simulink model "SF005A_StOutpCtrl"  (R2013b)
settings: Solver=FixedStepDiscrete  SolverMode=SingleTasking  StartTime=0.0  StopTime=1  FixedStep=0.002  RelTol=1e-3
values from neighbouring files (symbols this model uses):
  ARCHGLBPRM_2MILLISEC_SEC_F32 = DataDict.Constant    [SF005A_StOutpCtrl_DataDict.m]
  ARCHGLBPRM_FLOATZEROTHD_ULS_F32 = DataDict.Constant    [SF005A_StOutpCtrl_DataDict.m]
  BIGSLEW_ULSPERSEC_F32 = DataDict.Constant    [SF005A_StOutpCtrl_DataDict.m]
  DI_CNT_U08 = DataDict.Constant    [SF005A_StOutpCtrl_DataDict.m]
  LOA_CNT_U08 = DataDict.Constant    [SF005A_StOutpCtrl_DataDict.m]
  OPER_CNT_U08 = DataDict.Constant    [SF005A_StOutpCtrl_DataDict.m]
  STRTSTOP_CNT_U08 = DataDict.Constant    [SF005A_StOutpCtrl_DataDict.m]
libraries: NxtrLim x3, simulink x2
(part 1 of 2)
settings Model: Creator=lzz0tm  LastModifiedBy=FZG88Y
settings SolverCC: AutoInsertRateTranBlk=on  InsertRTBMode=Always
settings DataIOCC: LimitDataPoints=off  SaveFormat=Structure  ReturnWorkspaceOutputs=on
settings OptimizationCC: BlockReduction=off  InlineParams=on  ZeroExternalMemoryAtStartup=off  ZeroInternalMemoryAtStartup=off  OptimizeModelRefInitCode=on  LifeSpan=1
settings DebuggingCC: SignalInfNanChecking=error  SignalRangeChecking=warning  UnderspecifiedInitializationDetection=Simplified  SolverPrmCheckMsg=error  InheritedTsInSrcMsg=error  DiscreteInheritContinuousMsg=error  SingleTaskRateTransMsg=error  TasksWithSamePriorityMsg=error  SigSpecEnsureSampleTimeMsg=error  CheckMatrixSingularityMsg=error  ParameterUnderflowMsg=error  ParameterPrecisionLossMsg=error  ParameterTunabilityLossMsg=error  FixptConstUnderflowMsg=warning  FixptConstOverflowMsg=warning  VectorMatrixConversionMsg=error  SignalLabelMismatchMsg=error  UnconnectedInputMsg=error  UnconnectedOutputMsg=error  UnconnectedLineMsg=error  SFcnCompatibilityMsg=error  UniqueDataStoreMsg=warning  BusObjectLabelMismatch=error  RootOutportRequireBusObject=error  AssertControl=DisableAll  ModelReferenceIOMsg=error  ModelReferenceVersionMismatchMessage=warning  ModelReferenceIOMismatchMessage=error  ModelReferenceCSMismatchMessage=warning  ModelReferenceDataLoggingMessage=error  StateNameClashWarn=warning  StrictBusMsg=ErrorOnBusTreatedAsVector  NonBusSignalsTreatedAsBus=error  SFUnexpectedBacktrackingDiag=error  SFInvalidInputDataAccessInChartInitDiag=error  SFNoUnconditionalDefaultTransitionDiag=error  SFTransitionOutsideNaturalParentDiag=error  SFUnconditionalTransitionShadowingDiag=error  SFUndirectedBroadcastEventsDiag=error
settings ModelReferenceCC: ModelReferenceNumInstancesAllowed=Single
settings RTWCC: SystemTargetFile=autosar.tlc  GenCodeOnly=on  TemplateMakefile=ert_default_tmf  Description=AUTOSAR  GenerateReport=on  ProcessScript=autosar_make_rtw_hook  LaunchReport=on
settings CodeAppCC: GenerateComments=off  IgnoreCustomStorageClasses=off  CustomSymbolStrType=$N$R$M  CustomSymbolStrBlkIO=$N$M  SimulinkBlockComments=off
settings STFCustomTargetCC: ParMdlRefBuildCompliant=on  CompOptLevelCompliant=on  IncludeMdlTerminateFcn=off  CombineOutputUpdateFcns=on  SuppressErrorStatus=on  ERTFirstTimeCompliant=on  ERTCustomFileBanners=on  SupportNonFinite=off  SupportComplex=off  SupportContinuousTime=off  SupportNonInlinedSFcns=off  MATLABClassNameForMDSCustomization=Simulink.SoftwareTarget.ERTCustomization  AutosarCompliant=on  GRTInterface=off  SystemTargetFile=autosar.tlc
settings ERTTargetCC: CodeReplacementLibrary=ANSI_C  ConcurrentExecutionCompliant=off  IncludeMdlTerminateFcn=off  SuppressErrorStatus=on  SupportNonFinite=off  SupportComplex=off  ModelStepFunctionPrototypeControlCompliant=off  CPPClassGenCompliant=off  AutosarCompliant=on  InlinedParameterPlacement=NonHierarchical  ERTCustomFileTemplate=example_file_process.tlc  EnableUserReplacementTypes=on

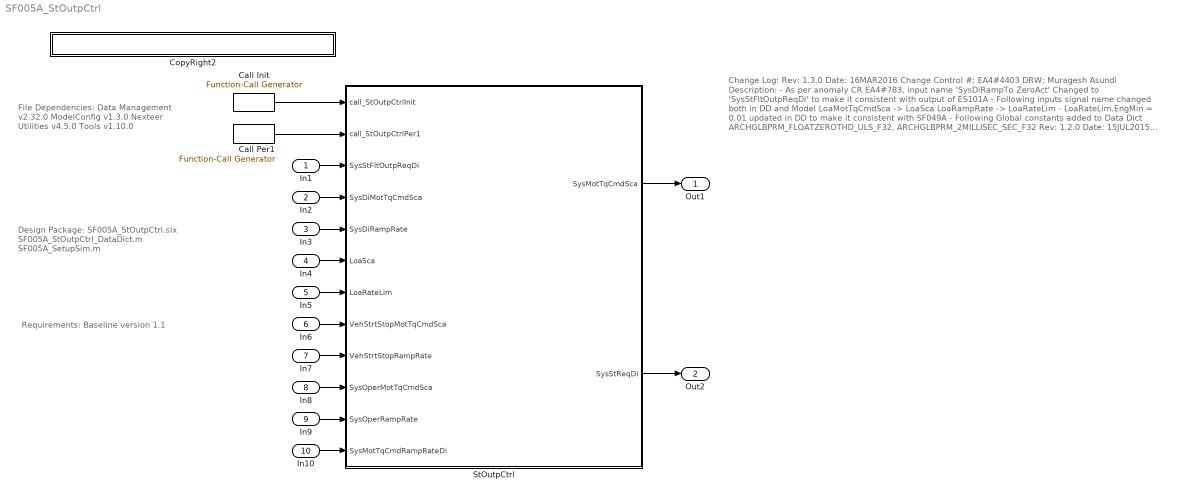
== system SF005A_StOutpCtrl ==
  note: Requirements: Baseline version 1.1
  note: Design Package:
      |
      | SF005A_StOutpCtrl.slx
      | SF005A_StOutpCtrl_DataDict.m
      | SF005A_SetupSim.m
  note: Change Log:
      |
      | Rev: 1.3.0
      | Date: 16MAR2016
      | Change Control #: EA4#4403
      | DRW: Muragesh Asundi
      | Description:
      | - As per anomaly CR EA4#783, input name 'SysDiRampTo ZeroAct'
      |  Changed to 'SysStFltOutpReqDi' to make it consistent with output of ES101A
      | - Following inputs signal name changed both in DD and Model
      |   LoaMotTqCmdSca -> LoaSca
      |   LoaRampRate -> LoaRateLim
      | - LoaRateLim.EngMin = 0.01 updated in DD to make it consistent with SF049A
      | - Following Global constants added to Data Dict
      |   ARCHGLBPRM_FLOATZEROTHD_ULS_F32,
      |   ARCHGLBPRM_2MILLISEC_SEC_F32
      |
      | Rev: 1.2.0
      | Date: 15JUL2015
      | Change Control #: EA4#1126
      | DRW: C. Wheatley
      | Description:
      | - EngInit values changed for:
      | 	LoaMotTqCmdSca
      | 	SysDiMotTqCmdSca
      | 	SysOperMotTqCmdSca
      | 	VehStrtStopMotTqCmdSca
      | 	SysMotTqCmdSca
      |
      | Rev: 1.1.0
      | Date: 22MAY2015
      | Change Control #:EA4#614
      | DRW: C. Wheatley
      | Description:
      | - StOutpCtrlInit renamed to StOutpCtrlInit1
      | - Constants used in the Init function
      | - Bug fixed in Target Selection function to handle
      |   an 'else' condition for state variable
      | - RATELIMITLO_ULSPERSEC_F32 value fixed
      |
      | Rev: 1.0.0
      | Date:30APR2015
      | Change Control #:EA4#521
      | DRW: C. Wheatley
      | Description:
      | - Initial release in EA4
      | - Based on Revision 4.0.0 in EA3
  note: File Dependencies:
      |
      | Data Management v2.32.0
      | ModelConfig v1.3.0
      | Nexteer Utilities v4.5.0
      | Tools v1.10.0
  In1 : Inport
  In2 : Inport  Port=2
  In3 : Inport  Port=3
  In4 : Inport  Port=4
  In5 : Inport  Port=5
  In6 : Inport  Port=6
  In7 : Inport  Port=7
  In8 : Inport  Port=8
  In9 : Inport  Port=9
  In10 : Inport  Port=10
  Call Init : simulink/Ports & Subsystems/Function-Call Generator  RequirementInfo={} %GIDa_fdbc255c_3555_4bfb_8d04_73a5fe8a9af7  sample_time=0.002  numberOfIterations=1
  Call Per1 : simulink/Ports & Subsystems/Function-Call Generator  RequirementInfo={} %GIDa_aefd7482_db29_41b3_b581_fef55ce184cb  sample_time=0.002  numberOfIterations=1
  CopyRight2 : Subsystem  Description=|  mask(Copyright Information){none=on}
      | Copyright info block.                                               
      |                                                                     
      | Place copyright information at the top of every subsystem in design.
      mask prompts: none "No parameters"
      mask help: Place copyright information at the top of every subsystem in design.
      mask Display:
      | NxtrConf = 'Nexteer Confidential';
      | 
      | sys = bdroot; %handle for the current model ("system")
      | first = get_param(sys,'Created');
      | first = first(end-3:end);  %year is last four digits
      | 
      | last = get_param(sys,'LastModifiedDate');
      | if isempty(last)
      |     last = datestr(now,'yyyy');
      | else
      |     last = last(end-3:end);
      | end
      | 
      | if strcmp(first,last)
      |     fprintf('%s -- Copyright %s Nexteer',NxtrConf,first)
      | else
      |     fprintf('%s -- %s%s- %s Nexteer',NxtrConf,char(169),first,last)
      | end
  StOutpCtrl : Subsystem  RequirementInfo={} %GIDa_19dfa550_9c7b_45b4_9a4a_0865bf4ef00b
  Out1 : Outport
  Out2 : Outport  Port=2
  wires:
  StOutpCtrl/1(SysMotTqCmdSca) -> Out1/1
  StOutpCtrl/2(SysStReqDi) -> Out2/1
  In1/1 -> StOutpCtrl/3(SysStFltOutpReqDi)
  In2/1 -> StOutpCtrl/4(SysDiMotTqCmdSca)
  In3/1 -> StOutpCtrl/5(SysDiRampRate)
  In4/1 -> StOutpCtrl/6(LoaSca)
  In5/1 -> StOutpCtrl/7(LoaRateLim)
  In6/1 -> StOutpCtrl/8(VehStrtStopMotTqCmdSca)
  In7/1 -> StOutpCtrl/9(VehStrtStopRampRate)
  In8/1 -> StOutpCtrl/10(SysOperMotTqCmdSca)
  In9/1 -> StOutpCtrl/11(SysOperRampRate)
  In10/1 -> StOutpCtrl/12(SysMotTqCmdRampRateDi)
  Call Per1/1 -> StOutpCtrl/2(call_StOutpCtrlPer1)
  Call Init/1 -> StOutpCtrl/1(call_StOutpCtrlInit)

== system SF005A_StOutpCtrl/CopyRight2 ==

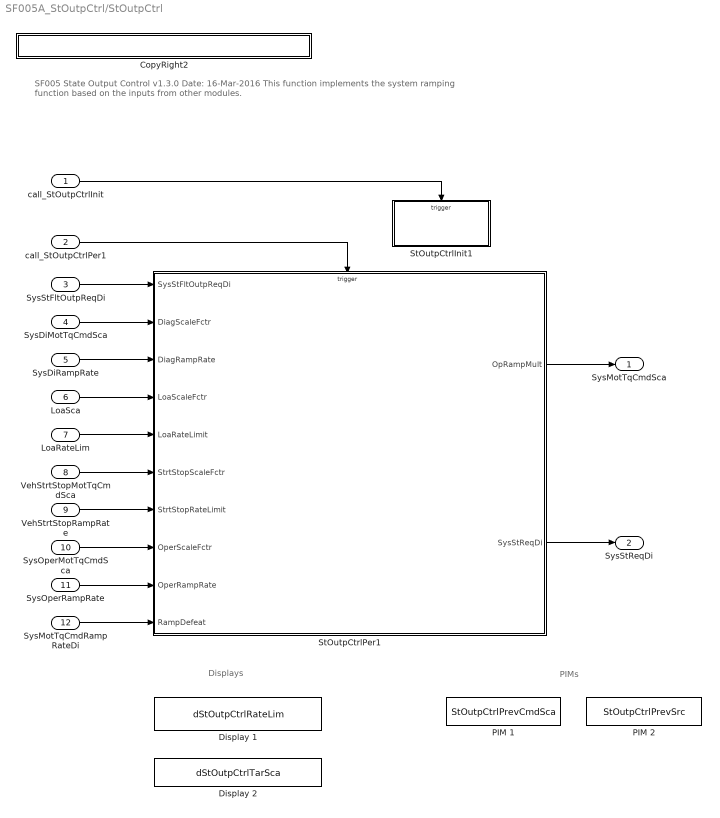
== system SF005A_StOutpCtrl/StOutpCtrl ==
  note: PIMs
  note: Displays
  note: SF005 State Output Control
      | v1.3.0 Date: 16-Mar-2016
      |
      | This function implements the system ramping function based on the inputs from other modules.
  call_StOutpCtrlInit : Inport
  call_StOutpCtrlPer1 : Inport  RequirementInfo={} %GIDa_d9bcf00b_26bb_4d5f_9706_6259ecb40bde  Port=2
  SysStFltOutpReqDi : Inport  RequirementInfo={'linktype_rmi_doors' '0000baae (/E-STEER Core/SubSystem Specifications/Application Functions/SF005A State Output Control)' '#SF005A_44' 'true' 'REQ: SF005A_44' '' } %GIDa_e055dff5_785c_40df_95c6_2dd67833b75a  Port=3
  SysDiMotTqCmdSca : Inport  RequirementInfo={'linktype_rmi_doors' '0000baae (/E-STEER Core/SubSystem Specifications/Application Functions/SF005A State Output Control)' '#SF005A_27' 'true' 'REQ: SF005A_27' '' } %GIDa_ef37b7cf_d2d5_4859_afe4_79c3a4ac5d62  Port=4
  SysDiRampRate : Inport  RequirementInfo={'linktype_rmi_doors' '0000baae (/E-STEER Core/SubSystem Specifications/Application Functions/SF005A State Output Control)' '#SF005A_36' 'true' 'REQ: SF005A_36' '' } %GIDa_75a2cdcb_c056_4580_94a8_b0d6a8309800  Port=5
  LoaSca : Inport  RequirementInfo={'linktype_rmi_doors' '0000baae (/E-STEER Core/SubSystem Specifications/Application Functions/SF005A State Output Control)' '#SF005A_37' 'true' 'REQ: SF005A_37' '' } %GIDa_7c52f51b_f85e_4c11_af12_dfe90bf6d347  Port=6
  LoaRateLim : Inport  RequirementInfo={'linktype_rmi_doors' '0000baae (/E-STEER Core/SubSystem Specifications/Application Functions/SF005A State Output Control)' '#SF005A_38' 'true' 'REQ: SF005A_38' '' } %GIDa_203dcbbb_c1e8_47f5_bd3f_ceea86e11bc3  Port=7
  VehStrtStopMotTqCmdSca : Inport  RequirementInfo={'linktype_rmi_doors' '0000baae (/E-STEER Core/SubSystem Specifications/Application Functions/SF005A State Output Control)' '#SF005A_39' 'true' 'REQ: SF005A_39' '' } %GIDa_4dfcc44e_73be_4632_bdf4_5443a534f587  Port=8
  VehStrtStopRampRate : Inport  RequirementInfo={'linktype_rmi_doors' '0000baae (/E-STEER Core/SubSystem Specifications/Application Functions/SF005A State Output Control)' '#SF005A_40' 'true' 'REQ: SF005A_40' '' } %GIDa_a84b4afb_5771_43dc_98ab_9288d1a52c0b  Port=9
  SysOperMotTqCmdSca : Inport  RequirementInfo={'linktype_rmi_doors' '0000baae (/E-STEER Core/SubSystem Specifications/Application Functions/SF005A State Output Control)' '#SF005A_41' 'true' 'REQ: SF005A_41' '' } %GIDa_60ad9967_90e0_4a11_957f_97f730e69c4f  Port=10
  SysOperRampRate : Inport  RequirementInfo={'linktype_rmi_doors' '0000baae (/E-STEER Core/SubSystem Specifications/Application Functions/SF005A State Output Control)' '#SF005A_42' 'true' 'REQ: SF005A_42' '' } %GIDa_aa5df56f_2a5c_44a8_8839_62b413ee5337  Port=11
  SysMotTqCmdRampRateDi : Inport  RequirementInfo={'linktype_rmi_doors' '0000baae (/E-STEER Core/SubSystem Specifications/Application Functions/SF005A State Output Control)' '#SF005A_43' 'true' 'REQ: SF005A_43' '' } %GIDa_34840cb7_9916_4187_a95f_369f75322225  Port=12
  CopyRight2 : Subsystem  Description=|  mask(Copyright Information){none=on}
      | Copyright info block.                                               
      |                                                                     
      | Place copyright information at the top of every subsystem in design.
      mask prompts: none "No parameters"
      mask help: Place copyright information at the top of every subsystem in design.
      mask Display:
      | NxtrConf = 'Nexteer Confidential';
      | 
      | sys = bdroot; %handle for the current model ("system")
      | first = get_param(sys,'Created');
      | first = first(end-3:end);  %year is last four digits
      | 
      | last = get_param(sys,'LastModifiedDate');
      | if isempty(last)
      |     last = datestr(now,'yyyy');
      | else
      |     last = last(end-3:end);
      | end
      | 
      | if strcmp(first,last)
      |     fprintf('%s -- Copyright %s Nexteer',NxtrConf,first)
      | else
      |     fprintf('%s -- %s%s- %s Nexteer',NxtrConf,char(169),first,last)
      | end
  Display 1 : DataStoreMemory  DataStoreName=dStOutpCtrlRateLim  ReadBeforeWriteMsg=warning  WriteAfterWriteMsg=warning  WriteAfterReadMsg=warning  StateMustResolveToSignalObject=on
  Display 2 : DataStoreMemory  DataStoreName=dStOutpCtrlTarSca  ReadBeforeWriteMsg=warning  WriteAfterWriteMsg=warning  WriteAfterReadMsg=warning  StateMustResolveToSignalObject=on
  PIM 1 : DataStoreMemory  RequirementInfo={} %GIDa_6af2038a_595d_4d64_91c6_8390e9ddce88  DataStoreName=StOutpCtrlPrevCmdSca  StateMustResolveToSignalObject=on
  PIM 2 : DataStoreMemory  RequirementInfo={} %GIDa_00d9f7bc_1c0b_4f19_a5e8_b9808d8978d9  DataStoreName=StOutpCtrlPrevSrc  StateMustResolveToSignalObject=on
  StOutpCtrlInit1 : Subsystem
  StOutpCtrlPer1 : Subsystem
  SysMotTqCmdSca : Outport  RequirementInfo={'linktype_rmi_doors' '0000baae (/E-STEER Core/SubSystem Specifications/Application Functions/SF005A State Output Control)' '#SF005A_28' 'true' 'REQ: SF005A_28' '' } %GIDa_033ab4ac_e16f_41c5_9cce_d2f08bd21db5
  SysStReqDi : Outport  RequirementInfo={'linktype_rmi_doors' '0000baae (/E-STEER Core/SubSystem Specifications/Application Functions/SF005A State Output Control)' '#SF005A_45' 'true' 'REQ: SF005A_45' '' } %GIDa_974dd383_3f68_4241_9569_44a3590de508  Port=2
  wires:
  SysStFltOutpReqDi/1 -> StOutpCtrlPer1/1(SysStFltOutpReqDi)
  SysDiMotTqCmdSca/1 -> StOutpCtrlPer1/2(DiagScaleFctr)
  SysDiRampRate/1 -> StOutpCtrlPer1/3(DiagRampRate)
  LoaSca/1 -> StOutpCtrlPer1/4(LoaScaleFctr)
  LoaRateLim/1 -> StOutpCtrlPer1/5(LoaRateLimit)
  VehStrtStopMotTqCmdSca/1 -> StOutpCtrlPer1/6(StrtStopScaleFctr)
  VehStrtStopRampRate/1 -> StOutpCtrlPer1/7(StrtStopRateLimit)
  SysOperMotTqCmdSca/1 -> StOutpCtrlPer1/8(OperScaleFctr)
  SysOperRampRate/1 -> StOutpCtrlPer1/9(OperRampRate)
  SysMotTqCmdRampRateDi/1 -> StOutpCtrlPer1/10(RampDefeat)
  StOutpCtrlPer1/1(OpRampMult) -> SysMotTqCmdSca/1
  StOutpCtrlPer1/2(SysStReqDi) -> SysStReqDi/1
  call_StOutpCtrlPer1/1 -> StOutpCtrlPer1/Trigger
  call_StOutpCtrlInit/1 -> StOutpCtrlInit1/Trigger

== system SF005A_StOutpCtrl/StOutpCtrl/CopyRight2 ==

== system SF005A_StOutpCtrl/StOutpCtrl/StOutpCtrlInit1 ==
  function : TriggerPort  TriggerType=function-call  PortDimensions=1
  Constant : Constant  Value=OPER_CNT_U08  OutDataTypeStr=uint8
  CopyRight2 : Subsystem  Description=|  mask(Copyright Information){none=on}
      | Copyright info block.                                               
      |                                                                     
      | Place copyright information at the top of every subsystem in design.
      mask prompts: none "No parameters"
      mask help: Place copyright information at the top of every subsystem in design.
      mask Display:
      | NxtrConf = 'Nexteer Confidential';
      | 
      | sys = bdroot; %handle for the current model ("system")
      | first = get_param(sys,'Created');
      | first = first(end-3:end);  %year is last four digits
      | 
      | last = get_param(sys,'LastModifiedDate');
      | if isempty(last)
      |     last = datestr(now,'yyyy');
      | else
      |     last = last(end-3:end);
      | end
      | 
      | if strcmp(first,last)
      |     fprintf('%s -- Copyright %s Nexteer',NxtrConf,first)
      | else
      |     fprintf('%s -- %s%s- %s Nexteer',NxtrConf,char(169),first,last)
      | end
  Data Store Write : DataStoreWrite  DataStoreName=StOutpCtrlPrevSrc
  wires:
  Constant/1 -> Data Store Write/1

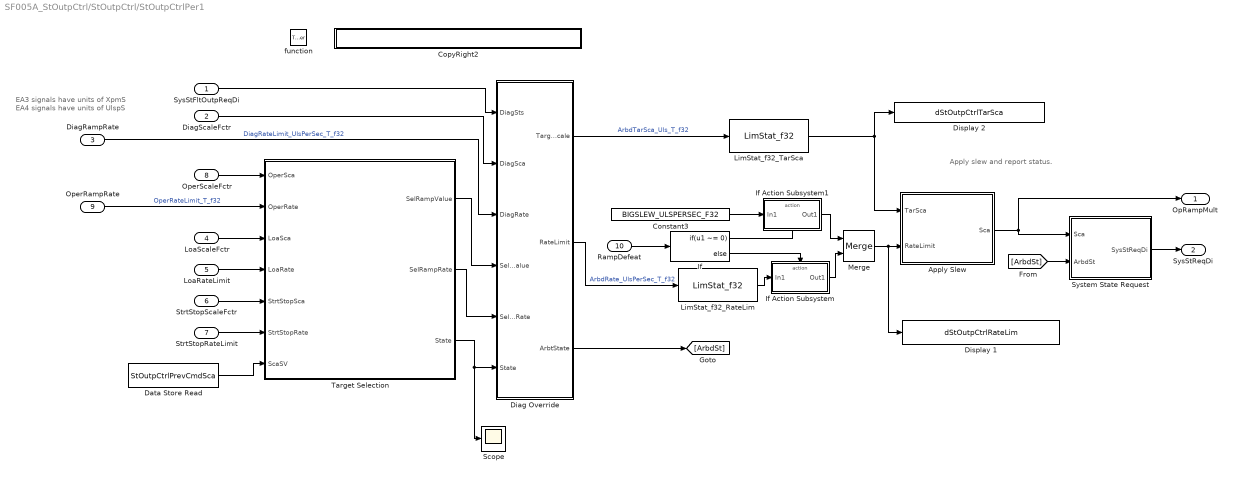
== system SF005A_StOutpCtrl/StOutpCtrl/StOutpCtrlPer1 ==
  note: EA3 signals have units of XpmS
      | EA4 signals have units of UlspS
  note: Apply slew and report status.
  SysStFltOutpReqDi : Inport
  DiagScaleFctr : Inport  Port=2
  DiagRampRate : Inport  Port=3
  LoaScaleFctr : Inport  Port=4
  LoaRateLimit : Inport  Port=5
  StrtStopScaleFctr : Inport  Port=6
  StrtStopRateLimit : Inport  Port=7
  OperScaleFctr : Inport  Port=8
  OperRampRate : Inport  Port=9
  RampDefeat : Inport  Port=10
  function : TriggerPort  TriggerType=function-call  PortDimensions=1
  Apply Slew : Subsystem  RequirementInfo={'linktype_rmi_doors' '0000baae (/E-STEER Core/SubSystem Specifications/Application Functions/SF005A State Output Control)' '#SF005A_57' 'true' 'REQ: SF005A_57' '' ; 'linktype_rmi_doors' '0000baae (/E-STEER Core/SubSystem Specifications/Application Functions/SF005A State Output Control)' '#SF005A_58' 'true' 'REQ: SF005A_58' '' } %GIDa_577a142a_c9f5_4151_a6a9_c77039d0532a
  Constant3 : Constant  RequirementInfo={'linktype_rmi_doors' '0000baae (/E-STEER Core/SubSystem Specifications/Application Functions/SF005A State Output Control)' '#SF005A_57' 'true' 'REQ: SF005A_57' '' } %GIDa_5f7830c5_5a04_4321_9058_a84341feb739  Value=BIGSLEW_ULSPERSEC_F32
  CopyRight2 : Subsystem  Description=|  mask(Copyright Information){none=on}
      | Copyright info block.                                               
      |                                                                     
      | Place copyright information at the top of every subsystem in design.
      mask prompts: none "No parameters"
      mask help: Place copyright information at the top of every subsystem in design.
      mask Display:
      | NxtrConf = 'Nexteer Confidential';
      | 
      | sys = bdroot; %handle for the current model ("system")
      | first = get_param(sys,'Created');
      | first = first(end-3:end);  %year is last four digits
      | 
      | last = get_param(sys,'LastModifiedDate');
      | if isempty(last)
      |     last = datestr(now,'yyyy');
      | else
      |     last = last(end-3:end);
      | end
      | 
      | if strcmp(first,last)
      |     fprintf('%s -- Copyright %s Nexteer',NxtrConf,first)
      | else
      |     fprintf('%s -- %s%s- %s Nexteer',NxtrConf,char(169),first,last)
      | end
  Data Store Read : DataStoreRead  DataStoreName=StOutpCtrlPrevCmdSca
  Diag Override : Subsystem  RequirementInfo={'linktype_rmi_doors' '0000baae (/E-STEER Core/SubSystem Specifications/Application Functions/SF005A State Output Control)' '#SF005A_50' 'true' 'REQ: SF005A_50' '' ; 'linktype_rmi_doors' '0000baae (/E-STEER Core/SubSystem Specifications/Application Functions/SF005A State Output Control)' '#SF005A_51' 'true' 'REQ: SF005A_51' '' } %GIDa_c251e99d_2666_46d6_9723_400adc1a8074
  Display 1 : DataStoreWrite  DataStoreName=dStOutpCtrlRateLim
  Display 2 : DataStoreWrite  DataStoreName=dStOutpCtrlTarSca
  If : If  IfExpression=u1 ~= 0
  If Action Subsystem : Subsystem  TreatAsAtomicUnit=on
  If Action Subsystem1 : Subsystem  TreatAsAtomicUnit=on
  LimStat_f32_RateLim : NxtrLim/LimStat_f32  RequirementInfo="{'linktype_rmi_doors' '0000baae (/E-STEER Core/SubSystem Specifications/Application Functions/SF005A State Output Control)' '#SF005A_69' 'true' 'REQ:  SF005A_69' '' } %GIDa_b1d99613_b57e_4c31_a899_1d75e103dc3b"  LoLim=RATELIMITLO_ULSPERSEC_F32  HiLim=RATELIMITHI_ULSPERSEC_F32
      settings: AttributesFormatString=|
      | Low Limit: %<LoLim>
      | High Limit: %<HiLim>
  LimStat_f32_TarSca : NxtrLim/LimStat_f32  RequirementInfo="{'linktype_rmi_doors' '0000baae (/E-STEER Core/SubSystem Specifications/Application Functions/SF005A State Output Control)' '#SF005A_68' 'true' 'REQ:  SF005A_68' '' } %GIDa_1b7cfcf7_e3e9_45d6_88ed_784366a66838"  LoLim=TARGETSCALELO_ULS_F32  HiLim=TARGETSCALEHI_ULS_F32
      settings: AttributesFormatString=|
      | Low Limit: %<LoLim>
      | High Limit: %<HiLim>
  Merge : Merge
  Scope : Scope
  "System State Request " : Subsystem  RequirementInfo={'linktype_rmi_doors' '0000baae (/E-STEER Core/SubSystem Specifications/Application Functions/SF005A State Output Control)' '#SF005A_60' 'true' 'REQ: SF005A_60' '' } %GIDa_c7536921_b563_4d8d_9444_00b81630476c
  Target Selection : Subsystem
  OpRampMult : Outport
  SysStReqDi : Outport  Port=2
  wires:
  Apply Slew/1(Sca) -> OpRampMult/1, "System State Request "/1(Sca)
  LoaScaleFctr/1 -> Target Selection/3(LoaSca)
  StrtStopScaleFctr/1 -> Target Selection/5(StrtStopSca)
  OperScaleFctr/1 -> Target Selection/1(OperSca)
  LoaRateLimit/1 -> Target Selection/4(LoaRate)
  StrtStopRateLimit/1 -> Target Selection/6(StrtStopRate)
  "System State Request "/1(SysStReqDi) -> SysStReqDi/1
  [ArbdSt] -> "System State Request "/2(ArbdSt)
  Diag Override/1(TargetScale) -> LimStat_f32_TarSca/1  "ArbdTarSca_Uls_T_f32"
  LimStat_f32_TarSca/1 -> Apply Slew/1(TarSca), Display 2/1
  Diag Override/2(RateLimit) -> LimStat_f32_RateLim/1  "ArbdRate_UlsPerSec_T_f32"
  OperRampRate/1 -> Target Selection/2(OperRate)  "OperRateLimit_T_f32"
  Data Store Read/1 -> Target Selection/7(ScaSV)
  If/1 -> If Action Subsystem1/Action
  If/2 -> If Action Subsystem/Action
  If Action Subsystem1/1(Out1) -> Merge/1
  If Action Subsystem/1(Out1) -> Merge/2
  Constant3/1 -> If Action Subsystem1/1(In1)
  Merge/1 -> Display 1/1, Apply Slew/2(RateLimit)
  RampDefeat/1 -> If/1
  LimStat_f32_RateLim/1 -> If Action Subsystem/1(In1)
  Target Selection/3(State) -> Scope/1, Diag Override/6(State)
  Target Selection/2(SelRampRate) -> Diag Override/5(SelRampRate)
  Target Selection/1(SelRampValue) -> Diag Override/4(SelRampValue)
  DiagRampRate/1 -> Diag Override/3(DiagRate)  "DiagRateLimit_UlsPerSec_T_f32"
  DiagScaleFctr/1 -> Diag Override/2(DiagSca)
  SysStFltOutpReqDi/1 -> Diag Override/1(DiagSts)
  Diag Override/3(ArbtState) -> [ArbdSt]

== system SF005A_StOutpCtrl/StOutpCtrl/StOutpCtrlInit1/CopyRight2 ==

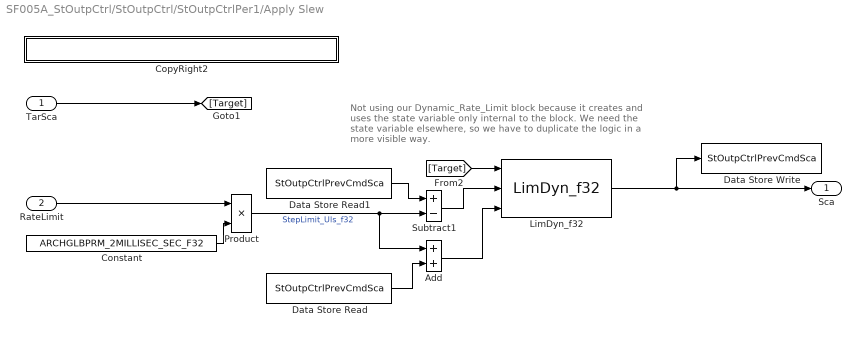
== system SF005A_StOutpCtrl/StOutpCtrl/StOutpCtrlPer1/Apply Slew ==
  note: Not using our Dynamic_Rate_Limit block because it creates
      | and uses the state variable only internal to the block.  We
      | need the state variable elsewhere, so we have to duplicate the
      | logic in a more visible way.
  TarSca : Inport
  RateLimit : Inport  Port=2
  Add : Sum
  Constant : Constant  RequirementInfo={'linktype_rmi_doors' '0000baae (/E-STEER Core/SubSystem Specifications/Application Functions/SF005A State Output Control)' '#SF005A_67' 'true' 'REQ: SF005A_67' '' } %GIDa_1bc3cf3d_97aa_4124_8be0_7f67e55dc7f2  Value=ARCHGLBPRM_2MILLISEC_SEC_F32
  CopyRight2 : Subsystem  Description=|  mask(Copyright Information){none=on}
      | Copyright info block.                                               
      |                                                                     
      | Place copyright information at the top of every subsystem in design.
      mask prompts: none "No parameters"
      mask help: Place copyright information at the top of every subsystem in design.
      mask Display:
      | NxtrConf = 'Nexteer Confidential';
      | 
      | sys = bdroot; %handle for the current model ("system")
      | first = get_param(sys,'Created');
      | first = first(end-3:end);  %year is last four digits
      | 
      | last = get_param(sys,'LastModifiedDate');
      | if isempty(last)
      |     last = datestr(now,'yyyy');
      | else
      |     last = last(end-3:end);
      | end
      | 
      | if strcmp(first,last)
      |     fprintf('%s -- Copyright %s Nexteer',NxtrConf,first)
      | else
      |     fprintf('%s -- %s%s- %s Nexteer',NxtrConf,char(169),first,last)
      | end
  Data Store Read : DataStoreRead  DataStoreName=StOutpCtrlPrevCmdSca
  Data Store Read1 : DataStoreRead  DataStoreName=StOutpCtrlPrevCmdSca
  Data Store Write : DataStoreWrite  DataStoreName=StOutpCtrlPrevCmdSca
  LimDyn_f32 : NxtrLim/LimDyn_f32
  Product : Product
  Subtract1 : Sum  Inputs=+-
  Sca : Outport
  wires:
  LimDyn_f32/1 -> Data Store Write/1, Sca/1
  TarSca/1 -> [Target]
  Data Store Read1/1 -> Subtract1/1
  RateLimit/1 -> Product/1
  Constant/1 -> Product/2
  Product/1 -> Add/1, Subtract1/2  "StepLimit_Uls_f32"
  [Target] -> LimDyn_f32/1
  Subtract1/1 -> LimDyn_f32/2
  Add/1 -> LimDyn_f32/3
  Data Store Read/1 -> Add/2

== system SF005A_StOutpCtrl/StOutpCtrl/StOutpCtrlPer1/CopyRight2 ==

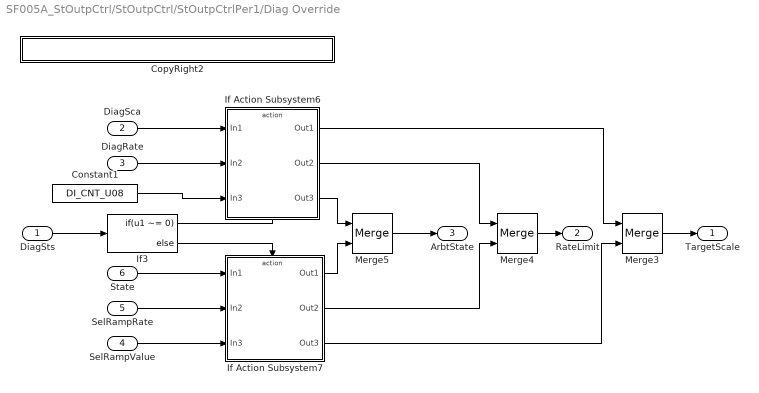
== system SF005A_StOutpCtrl/StOutpCtrl/StOutpCtrlPer1/Diag Override ==
  DiagSts : Inport
  DiagSca : Inport  Port=2
  DiagRate : Inport  Port=3
  SelRampValue : Inport  Port=4
  SelRampRate : Inport  Port=5
  State : Inport  Port=6
  Constant1 : Constant  Value=DI_CNT_U08  OutDataTypeStr=uint8
  CopyRight2 : Subsystem  Description=|  mask(Copyright Information){none=on}
      | Copyright info block.                                               
      |                                                                     
      | Place copyright information at the top of every subsystem in design.
      mask prompts: none "No parameters"
      mask help: Place copyright information at the top of every subsystem in design.
      mask Display:
      | NxtrConf = 'Nexteer Confidential';
      | 
      | sys = bdroot; %handle for the current model ("system")
      | first = get_param(sys,'Created');
      | first = first(end-3:end);  %year is last four digits
      | 
      | last = get_param(sys,'LastModifiedDate');
      | if isempty(last)
      |     last = datestr(now,'yyyy');
      | else
      |     last = last(end-3:end);
      | end
      | 
      | if strcmp(first,last)
      |     fprintf('%s -- Copyright %s Nexteer',NxtrConf,first)
      | else
      |     fprintf('%s -- %s%s- %s Nexteer',NxtrConf,char(169),first,last)
      | end
  If Action Subsystem6 : Subsystem  TreatAsAtomicUnit=on
  If Action Subsystem7 : Subsystem  TreatAsAtomicUnit=on
  If3 : If  IfExpression=u1 ~= 0
  Merge3 : Merge
  Merge4 : Merge
  Merge5 : Merge
  TargetScale : Outport
  RateLimit : Outport  Port=2
  ArbtState : Outport  Port=3
  wires:
  If3/1 -> If Action Subsystem6/Action
  If3/2 -> If Action Subsystem7/Action
  If Action Subsystem6/1(Out1) -> Merge3/1
  Constant1/1 -> If Action Subsystem6/3(In3)
  If Action Subsystem6/3(Out3) -> Merge5/1
  If Action Subsystem6/2(Out2) -> Merge4/1
  Merge3/1 -> TargetScale/1
  Merge4/1 -> RateLimit/1
  Merge5/1 -> ArbtState/1
  SelRampRate/1 -> If Action Subsystem7/2(In2)
  DiagRate/1 -> If Action Subsystem6/2(In2)
  DiagSca/1 -> If Action Subsystem6/1(In1)
  DiagSts/1 -> If3/1
  If Action Subsystem7/1(Out1) -> Merge5/2
  If Action Subsystem7/2(Out2) -> Merge4/2
  If Action Subsystem7/3(Out3) -> Merge3/2
  State/1 -> If Action Subsystem7/1(In1)
  SelRampValue/1 -> If Action Subsystem7/3(In3)

== system SF005A_StOutpCtrl/StOutpCtrl/StOutpCtrlPer1/If Action Subsystem ==
  In1 : Inport
  Action Port : ActionPort  ActionType=else
  Out1 : Outport
  wires:
  In1/1 -> Out1/1

== system SF005A_StOutpCtrl/StOutpCtrl/StOutpCtrlPer1/If Action Subsystem1 ==
  In1 : Inport
  Action Port : ActionPort  ActionType=then
  Out1 : Outport
  wires:
  In1/1 -> Out1/1

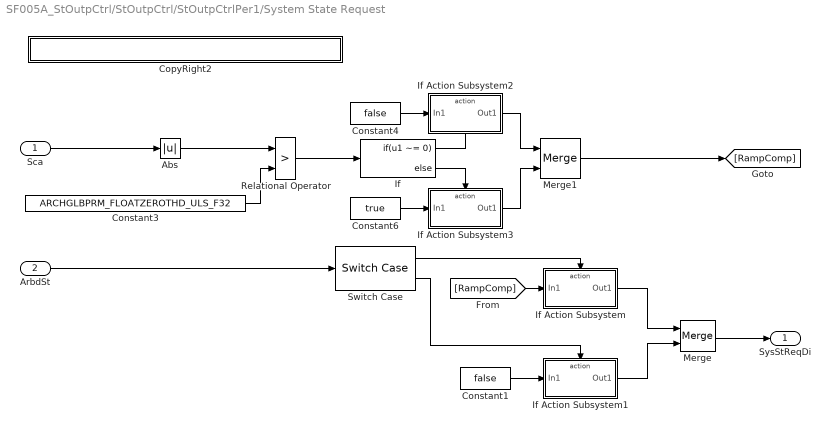
== system SF005A_StOutpCtrl/StOutpCtrl/StOutpCtrlPer1/System State Request  ==
  Sca : Inport
  ArbdSt : Inport  Port=2
  Abs : Abs
  Constant1 : Constant  Value=false
  Constant3 : Constant  Value=ARCHGLBPRM_FLOATZEROTHD_ULS_F32
  Constant4 : Constant  Value=false
  Constant6 : Constant  Value=true
  CopyRight2 : Subsystem  Description=|  mask(Copyright Information){none=on}
      | Copyright info block.                                               
      |                                                                     
      | Place copyright information at the top of every subsystem in design.
      mask prompts: none "No parameters"
      mask help: Place copyright information at the top of every subsystem in design.
      mask Display:
      | NxtrConf = 'Nexteer Confidential';
      | 
      | sys = bdroot; %handle for the current model ("system")
      | first = get_param(sys,'Created');
      | first = first(end-3:end);  %year is last four digits
      | 
      | last = get_param(sys,'LastModifiedDate');
      | if isempty(last)
      |     last = datestr(now,'yyyy');
      | else
      |     last = last(end-3:end);
      | end
      | 
      | if strcmp(first,last)
      |     fprintf('%s -- Copyright %s Nexteer',NxtrConf,first)
      | else
      |     fprintf('%s -- %s%s- %s Nexteer',NxtrConf,char(169),first,last)
      | end
  If : If  IfExpression=u1 ~= 0
  If Action Subsystem : Subsystem  TreatAsAtomicUnit=on
  If Action Subsystem1 : Subsystem  TreatAsAtomicUnit=on
  If Action Subsystem2 : Subsystem  TreatAsAtomicUnit=on
  If Action Subsystem3 : Subsystem  TreatAsAtomicUnit=on
  Merge : Merge
  Merge1 : Merge
  Relational Operator : RelationalOperator  Operator=>  OutDataTypeStr=boolean
  Switch Case : SwitchCase  CaseConditions={[1,4]}
  SysStReqDi : Outport
  wires:
  Abs/1 -> Relational Operator/1
  Constant3/1 -> Relational Operator/2
  Sca/1 -> Abs/1
  Switch Case/1 -> If Action Subsystem/Action
  [RampComp] -> If Action Subsystem/1(In1)
  Switch Case/2 -> If Action Subsystem1/Action
  Constant1/1 -> If Action Subsystem1/1(In1)
  Merge/1 -> SysStReqDi/1
  If Action Subsystem/1(Out1) -> Merge/1
  If Action Subsystem1/1(Out1) -> Merge/2
  ArbdSt/1 -> Switch Case/1
  If/2 -> If Action Subsystem3/Action
  If/1 -> If Action Subsystem2/Action
  If Action Subsystem2/1(Out1) -> Merge1/1
  If Action Subsystem3/1(Out1) -> Merge1/2
  Constant4/1 -> If Action Subsystem2/1(In1)
  Constant6/1 -> If Action Subsystem3/1(In1)
  Relational Operator/1 -> If/1
  Merge1/1 -> [RampComp]

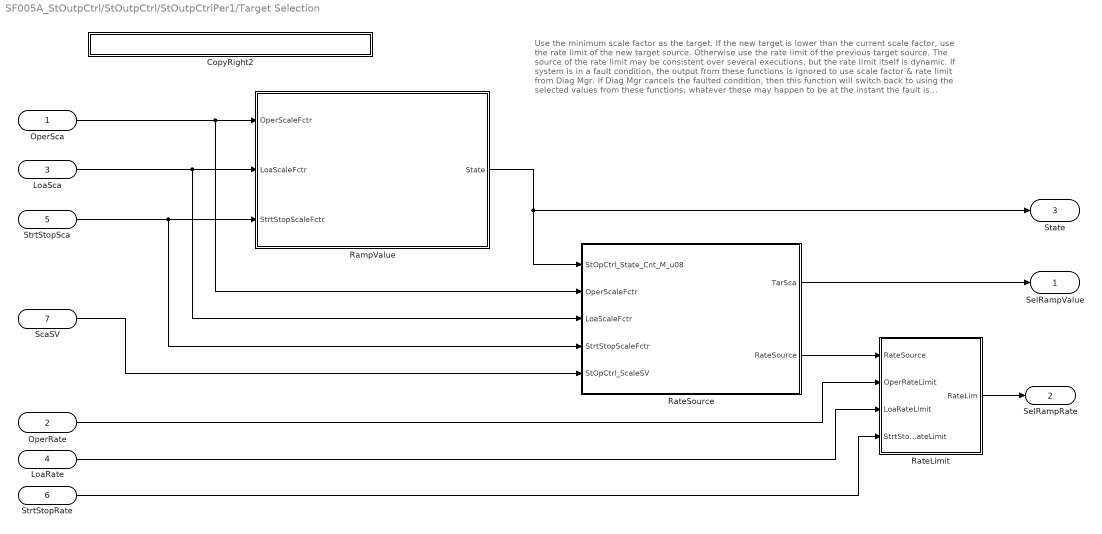
== system SF005A_StOutpCtrl/StOutpCtrl/StOutpCtrlPer1/Target Selection ==
  note: Use the minimum scale factor as the target. If the new target is lower than the current scale factor,
      | use the rate limit of the new target source.  Otherwise use the rate limit of the previous target source.
      | The source of the rate limit may be consistent over several executions, but the rate limit itself is dynamic.
      |
      | If system is in a fault condition, the output from these functions is ignored to use scale factor & rate limit from Diag Mgr.
      | If Diag Mgr cancels the faulted condition, then this function will switch back to using the selected values from these functions;
      | whatever those may happen to be at the instant the fault is cancelled.
  OperSca : Inport  RequirementInfo={} %GIDa_849c9a87_8d03_4e64_a43d_051ae1b79f36
  OperRate : Inport  Port=2
  LoaSca : Inport  Port=3
  LoaRate : Inport  Port=4
  StrtStopSca : Inport  Port=5
  StrtStopRate : Inport  Port=6
  ScaSV : Inport  Port=7
  CopyRight2 : Subsystem  Description=|  mask(Copyright Information){none=on}
      | Copyright info block.                                               
      |                                                                     
      | Place copyright information at the top of every subsystem in design.
      mask prompts: none "No parameters"
      mask help: Place copyright information at the top of every subsystem in design.
      mask Display:
      | NxtrConf = 'Nexteer Confidential';
      | 
      | sys = bdroot; %handle for the current model ("system")
      | first = get_param(sys,'Created');
      | first = first(end-3:end);  %year is last four digits
      | 
      | last = get_param(sys,'LastModifiedDate');
      | if isempty(last)
      |     last = datestr(now,'yyyy');
      | else
      |     last = last(end-3:end);
      | end
      | 
      | if strcmp(first,last)
      |     fprintf('%s -- Copyright %s Nexteer',NxtrConf,first)
      | else
      |     fprintf('%s -- %s%s- %s Nexteer',NxtrConf,char(169),first,last)
      | end
  RampValue : Subsystem  RequirementInfo={'linktype_rmi_doors' '0000baae (/E-STEER Core/SubSystem Specifications/Application Functions/SF005A State Output Control)' '#SF005A_52' 'true' 'REQ: SF005A_52' '' } %GIDa_541aa908_ad23_4d91_ad3b_86296622d1df
  RateLimit : Subsystem  RequirementInfo={'linktype_rmi_doors' '0000baae (/E-STEER Core/SubSystem Specifications/Application Functions/SF005A State Output Control)' '#SF005A_53' 'true' 'REQ: SF005A_53' '' } %GIDa_532f313a_08a5_4c70_9503_e8ee6a10fd80
  RateSource : Subsystem
  SelRampValue : Outport
  SelRampRate : Outport  Port=2
  State : Outport  Port=3
  wires:
  RateSource/1(TarSca) -> SelRampValue/1
  StrtStopRate/1 -> RateLimit/4(StrtStopRateLimit)
  LoaRate/1 -> RateLimit/3(LoaRateLimit)
  OperRate/1 -> RateLimit/2(OperRateLimit)
  RateSource/2(RateSource) -> RateLimit/1(RateSource)
  RateLimit/1(RateLim) -> SelRampRate/1
  ScaSV/1 -> RateSource/5(StOpCtrl_ScaleSV)
  RampValue/1(State) -> RateSource/1(StOpCtrl_State_Cnt_M_u08), State/1
  OperSca/1 -> RampValue/1(OperScaleFctr), RateSource/2(OperScaleFctr)
  StrtStopSca/1 -> RampValue/3(StrtStopScaleFctr), RateSource/4(StrtStopScaleFctr)
  LoaSca/1 -> RampValue/2(LoaScaleFctr), RateSource/3(LoaScaleFctr)

== system SF005A_StOutpCtrl/StOutpCtrl/StOutpCtrlPer1/Apply Slew/CopyRight2 ==

== system SF005A_StOutpCtrl/StOutpCtrl/StOutpCtrlPer1/Diag Override/CopyRight2 ==

== system SF005A_StOutpCtrl/StOutpCtrl/StOutpCtrlPer1/Diag Override/If Action Subsystem6 ==
  In1 : Inport
  In2 : Inport  Port=2
  In3 : Inport  Port=3
  Action Port : ActionPort  ActionType=then
  Out1 : Outport
  Out2 : Outport  Port=2
  Out3 : Outport  Port=3
  wires:
  In1/1 -> Out1/1
  In2/1 -> Out2/1
  In3/1 -> Out3/1

== system SF005A_StOutpCtrl/StOutpCtrl/StOutpCtrlPer1/Diag Override/If Action Subsystem7 ==
  In1 : Inport
  In2 : Inport  Port=2
  In3 : Inport  Port=3
  Action Port : ActionPort  ActionType=else
  Out1 : Outport
  Out2 : Outport  Port=2
  Out3 : Outport  Port=3
  wires:
  In1/1 -> Out1/1
  In2/1 -> Out2/1
  In3/1 -> Out3/1

== system SF005A_StOutpCtrl/StOutpCtrl/StOutpCtrlPer1/System State Request /CopyRight2 ==

== system SF005A_StOutpCtrl/StOutpCtrl/StOutpCtrlPer1/System State Request /If Action Subsystem ==
  In1 : Inport
  Action Port : ActionPort  ActionType=case
  Out1 : Outport
  wires:
  In1/1 -> Out1/1

== system SF005A_StOutpCtrl/StOutpCtrl/StOutpCtrlPer1/System State Request /If Action Subsystem1 ==
  In1 : Inport
  Action Port : ActionPort  ActionType=default
  Out1 : Outport
  wires:
  In1/1 -> Out1/1

== system SF005A_StOutpCtrl/StOutpCtrl/StOutpCtrlPer1/System State Request /If Action Subsystem2 ==
  In1 : Inport
  Action Port : ActionPort  ActionType=then
  Out1 : Outport
  wires:
  In1/1 -> Out1/1

== system SF005A_StOutpCtrl/StOutpCtrl/StOutpCtrlPer1/System State Request /If Action Subsystem3 ==
  In1 : Inport
  Action Port : ActionPort  ActionType=else
  Out1 : Outport
  wires:
  In1/1 -> Out1/1

== system SF005A_StOutpCtrl/StOutpCtrl/StOutpCtrlPer1/Target Selection/CopyRight2 ==

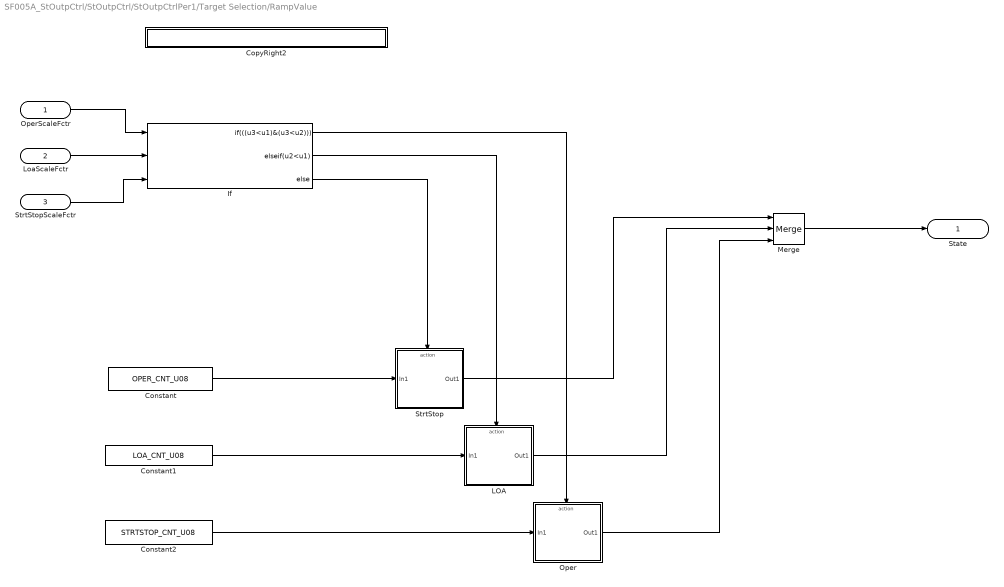
== system SF005A_StOutpCtrl/StOutpCtrl/StOutpCtrlPer1/Target Selection/RampValue ==
  OperScaleFctr : Inport
  LoaScaleFctr : Inport  Port=2
  StrtStopScaleFctr : Inport  Port=3
  Constant : Constant  Value=OPER_CNT_U08
  Constant1 : Constant  Value=LOA_CNT_U08
  Constant2 : Constant  Value=STRTSTOP_CNT_U08
  CopyRight2 : Subsystem  Description=|  mask(Copyright Information){none=on}
      | Copyright info block.                                               
      |                                                                     
      | Place copyright information at the top of every subsystem in design.
      mask prompts: none "No parameters"
      mask help: Place copyright information at the top of every subsystem in design.
      mask Display:
      | NxtrConf = 'Nexteer Confidential';
      | 
      | sys = bdroot; %handle for the current model ("system")
      | first = get_param(sys,'Created');
      | first = first(end-3:end);  %year is last four digits
      | 
      | last = get_param(sys,'LastModifiedDate');
      | if isempty(last)
      |     last = datestr(now,'yyyy');
      | else
      |     last = last(end-3:end);
      | end
      | 
      | if strcmp(first,last)
      |     fprintf('%s -- Copyright %s Nexteer',NxtrConf,first)
      | else
      |     fprintf('%s -- %s%s- %s Nexteer',NxtrConf,char(169),first,last)
      | end
  If : If  NumInputs=3  IfExpression=((u3<u1)&(u3<u2))  ElseIfExpressions=u2<u1
      settings: AttributesFormatString=|
      | if: ((u3<u1)&(u3<u2))
      | elseif: (u2<u1)
      | else:
  LOA : Subsystem  TreatAsAtomicUnit=on
  Merge : Merge  Inputs=3
  Oper : Subsystem  TreatAsAtomicUnit=on
  StrtStop : Subsystem  TreatAsAtomicUnit=on
  State : Outport
  wires:
  Oper/1(Out1) -> Merge/3
  LOA/1(Out1) -> Merge/2
  StrtStop/1(Out1) -> Merge/1
  StrtStopScaleFctr/1 -> If/3
  LoaScaleFctr/1 -> If/2
  OperScaleFctr/1 -> If/1
  If/2 -> LOA/Action
  If/3 -> StrtStop/Action
  Merge/1 -> State/1
  Constant1/1 -> LOA/1(In1)
  If/1 -> Oper/Action
  Constant/1 -> StrtStop/1(In1)
  Constant2/1 -> Oper/1(In1)

== system SF005A_StOutpCtrl/StOutpCtrl/StOutpCtrlPer1/Target Selection/RateLimit ==
  RateSource : Inport
  OperRateLimit : Inport  Port=2
  LoaRateLimit : Inport  Port=3
  StrtStopRateLimit : Inport  Port=4
  CopyRight2 : Subsystem  Description=|  mask(Copyright Information){none=on}
      | Copyright info block.                                               
      |                                                                     
      | Place copyright information at the top of every subsystem in design.
      mask prompts: none "No parameters"
      mask help: Place copyright information at the top of every subsystem in design.
      mask Display:
      | NxtrConf = 'Nexteer Confidential';
      | 
      | sys = bdroot; %handle for the current model ("system")
      | first = get_param(sys,'Created');
      | first = first(end-3:end);  %year is last four digits
      | 
      | last = get_param(sys,'LastModifiedDate');
      | if isempty(last)
      |     last = datestr(now,'yyyy');
      | else
      |     last = last(end-3:end);
      | end
      | 
      | if strcmp(first,last)
      |     fprintf('%s -- Copyright %s Nexteer',NxtrConf,first)
      | else
      |     fprintf('%s -- %s%s- %s Nexteer',NxtrConf,char(169),first,last)
      | end
  Loa : Subsystem  TreatAsAtomicUnit=on
  Merge : Merge  Inputs=3
  Oper : Subsystem  TreatAsAtomicUnit=on
  StrtStop : Subsystem  TreatAsAtomicUnit=on
  Switch Case : SwitchCase  CaseConditions={1,2,3}  ShowDefaultCase=off
      settings: AttributesFormatString=|
      | Case 1: Oper
      | Case 2: Loa
      | Case 3: StrtStop
  RateLim : Outport
  wires:
  RateSource/1 -> Switch Case/1
  OperRateLimit/1 -> Oper/1(In1)
  StrtStopRateLimit/1 -> StrtStop/1(In1)
  Merge/1 -> RateLim/1
  StrtStop/1(Out1) -> Merge/1
  Loa/1(Out1) -> Merge/2
  LoaRateLimit/1 -> Loa/1(In1)
  Switch Case/1 -> Oper/Action
  Switch Case/2 -> Loa/Action
  Switch Case/3 -> StrtStop/Action
  Oper/1(Out1) -> Merge/3

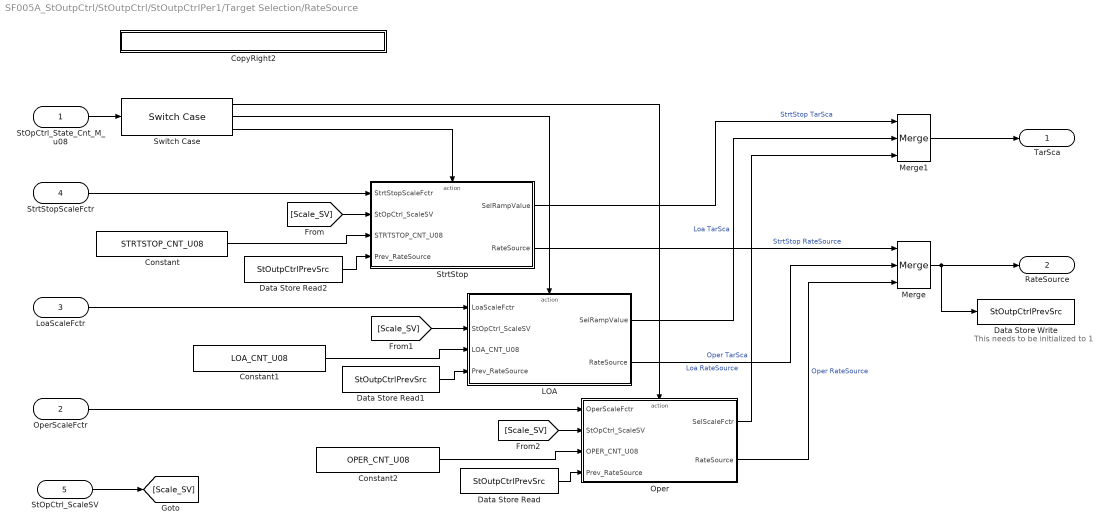
== system SF005A_StOutpCtrl/StOutpCtrl/StOutpCtrlPer1/Target Selection/RateSource ==
  note: This needs to be initialized to 1
  StOpCtrl_State_Cnt_M_u08 : Inport
  OperScaleFctr : Inport  Port=2
  LoaScaleFctr : Inport  Port=3
  StrtStopScaleFctr : Inport  Port=4
  StOpCtrl_ScaleSV : Inport  Port=5
  Constant : Constant  Value=STRTSTOP_CNT_U08
  Constant1 : Constant  Value=LOA_CNT_U08
  Constant2 : Constant  Value=OPER_CNT_U08
  CopyRight2 : Subsystem  Description=|  mask(Copyright Information){none=on}
      | Copyright info block.                                               
      |                                                                     
      | Place copyright information at the top of every subsystem in design.
      mask prompts: none "No parameters"
      mask help: Place copyright information at the top of every subsystem in design.
      mask Display:
      | NxtrConf = 'Nexteer Confidential';
      | 
      | sys = bdroot; %handle for the current model ("system")
      | first = get_param(sys,'Created');
      | first = first(end-3:end);  %year is last four digits
      | 
      | last = get_param(sys,'LastModifiedDate');
      | if isempty(last)
      |     last = datestr(now,'yyyy');
      | else
      |     last = last(end-3:end);
      | end
      | 
      | if strcmp(first,last)
      |     fprintf('%s -- Copyright %s Nexteer',NxtrConf,first)
      | else
      |     fprintf('%s -- %s%s- %s Nexteer',NxtrConf,char(169),first,last)
      | end
  Data Store Read : DataStoreRead  DataStoreName=StOutpCtrlPrevSrc
  Data Store Read1 : DataStoreRead  DataStoreName=StOutpCtrlPrevSrc
  Data Store Read2 : DataStoreRead  DataStoreName=StOutpCtrlPrevSrc
  Data Store Write : DataStoreWrite  DataStoreName=StOutpCtrlPrevSrc
  LOA : Subsystem
  Merge : Merge  Inputs=3
  Merge1 : Merge  Inputs=3
  Oper : Subsystem
  StrtStop : Subsystem
  Switch Case : SwitchCase  CaseConditions={1,2,3}  ShowDefaultCase=off
      settings: AttributesFormatString=|
      | case 1: Oper
      | case 2: Loa
      | case 3: StrtStop
  TarSca : Outport
  RateSource : Outport  Port=2
  wires:
  Merge1/1 -> TarSca/1
  Oper/1(SelScaleFctr) -> Merge1/3  "Oper TarSca"
  LOA/2(RateSource) -> Merge/2  "Loa RateSource"
  LOA/1(SelRampValue) -> Merge1/2  "Loa TarSca"
  StrtStop/1(SelRampValue) -> Merge1/1  "StrtStop TarSca"
  Constant/1 -> StrtStop/3(STRTSTOP_CNT_U08)
  Switch Case/1 -> Oper/Action
  Switch Case/2 -> LOA/Action
  Switch Case/3 -> StrtStop/Action
  Data Store Read2/1 -> StrtStop/4(Prev_RateSource)
  Data Store Read1/1 -> LOA/4(Prev_RateSource)
  [Scale_SV] -> Oper/2(StOpCtrl_ScaleSV)
  [Scale_SV] -> LOA/2(StOpCtrl_ScaleSV)
  [Scale_SV] -> StrtStop/2(StOpCtrl_ScaleSV)
  StOpCtrl_ScaleSV/1 -> [Scale_SV]
  StOpCtrl_State_Cnt_M_u08/1 -> Switch Case/1
  Constant2/1 -> Oper/3(OPER_CNT_U08)
  Constant1/1 -> LOA/3(LOA_CNT_U08)
  Oper/2(RateSource) -> Merge/3  "Oper RateSource"
  StrtStop/2(RateSource) -> Merge/1  "StrtStop RateSource"
  Merge/1 -> Data Store Write/1, RateSource/1
  StrtStopScaleFctr/1 -> StrtStop/1(StrtStopScaleFctr)
  OperScaleFctr/1 -> Oper/1(OperScaleFctr)
  LoaScaleFctr/1 -> LOA/1(LoaScaleFctr)
  Data Store Read/1 -> Oper/4(Prev_RateSource)

== system SF005A_StOutpCtrl/StOutpCtrl/StOutpCtrlPer1/Target Selection/RampValue/CopyRight2 ==

== system SF005A_StOutpCtrl/StOutpCtrl/StOutpCtrlPer1/Target Selection/RampValue/LOA ==
  In1 : Inport
  Action Port : ActionPort  ActionType=elseif
  Out1 : Outport
  wires:
  In1/1 -> Out1/1

== system SF005A_StOutpCtrl/StOutpCtrl/StOutpCtrlPer1/Target Selection/RampValue/Oper ==
  In1 : Inport
  Action Port : ActionPort  ActionType=then
  Out1 : Outport
  wires:
  In1/1 -> Out1/1

== system SF005A_StOutpCtrl/StOutpCtrl/StOutpCtrlPer1/Target Selection/RampValue/StrtStop ==
  In1 : Inport
  Action Port : ActionPort  ActionType=else
  Out1 : Outport
  wires:
  In1/1 -> Out1/1

== system SF005A_StOutpCtrl/StOutpCtrl/StOutpCtrlPer1/Target Selection/RateLimit/CopyRight2 ==

== system SF005A_StOutpCtrl/StOutpCtrl/StOutpCtrlPer1/Target Selection/RateLimit/Loa ==
  In1 : Inport
  Action Port : ActionPort  ActionType=case
  Out1 : Outport
  wires:
  In1/1 -> Out1/1

== system SF005A_StOutpCtrl/StOutpCtrl/StOutpCtrlPer1/Target Selection/RateLimit/Oper ==
  In1 : Inport
  Action Port : ActionPort  ActionType=case
  Out1 : Outport
  wires:
  In1/1 -> Out1/1

== system SF005A_StOutpCtrl/StOutpCtrl/StOutpCtrlPer1/Target Selection/RateLimit/StrtStop ==
  In1 : Inport
  Action Port : ActionPort  ActionType=case
  Out1 : Outport
  wires:
  In1/1 -> Out1/1

== system SF005A_StOutpCtrl/StOutpCtrl/StOutpCtrlPer1/Target Selection/RateSource/CopyRight2 ==

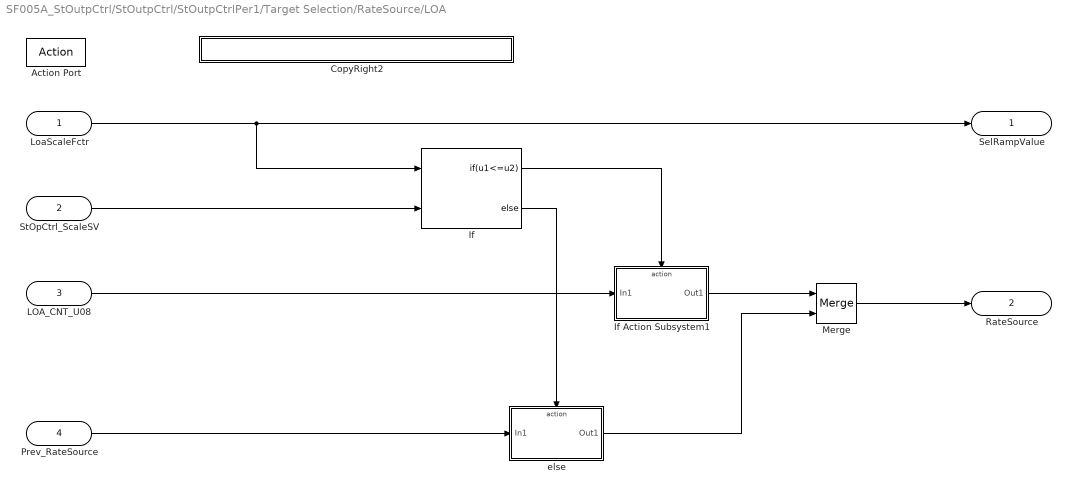
== system SF005A_StOutpCtrl/StOutpCtrl/StOutpCtrlPer1/Target Selection/RateSource/LOA ==
  LoaScaleFctr : Inport
  StOpCtrl_ScaleSV : Inport  Port=2
  LOA_CNT_U08 : Inport  Port=3
  Prev_RateSource : Inport  Port=4
  Action Port : ActionPort  ActionType=case
  CopyRight2 : Subsystem  Description=|  mask(Copyright Information){none=on}
      | Copyright info block.                                               
      |                                                                     
      | Place copyright information at the top of every subsystem in design.
      mask prompts: none "No parameters"
      mask help: Place copyright information at the top of every subsystem in design.
      mask Display:
      | NxtrConf = 'Nexteer Confidential';
      | 
      | sys = bdroot; %handle for the current model ("system")
      | first = get_param(sys,'Created');
      | first = first(end-3:end);  %year is last four digits
      | 
      | last = get_param(sys,'LastModifiedDate');
      | if isempty(last)
      |     last = datestr(now,'yyyy');
      | else
      |     last = last(end-3:end);
      | end
      | 
      | if strcmp(first,last)
      |     fprintf('%s -- Copyright %s Nexteer',NxtrConf,first)
      | else
      |     fprintf('%s -- %s%s- %s Nexteer',NxtrConf,char(169),first,last)
      | end
  If : If  RequirementInfo={'linktype_rmi_doors' '0000baae (/E-STEER Core/SubSystem Specifications/Application Functions/SF005A State Output Control)' '#SF005A_54' 'true' 'REQ: SF005A_54' '' ; 'linktype_rmi_doors' '0000baae (/E-STEER Core/SubSystem Specifications/Application Functions/SF005A State Output Control)' '#SF005A_55' 'true' 'REQ: SF005A_55' '' ; 'linktype_rmi_doors' '0000baae (/E-STEER Core/SubSystem Specifications/Application Functions/SF005A State Output Control)' '#SF005A_61' 'true' 'REQ: SF005A_61' '' } %GIDa_5c692240_752d_457b_a676_1ce9a35b4c5b  NumInputs=2  IfExpression=u1<=u2
  If Action Subsystem1 : Subsystem  TreatAsAtomicUnit=on
  Merge : Merge
  else : Subsystem  TreatAsAtomicUnit=on
  SelRampValue : Outport
  RateSource : Outport  Port=2
  wires:
  If Action Subsystem1/1(Out1) -> Merge/1
  else/1(Out1) -> Merge/2
  Merge/1 -> RateSource/1
  Prev_RateSource/1 -> else/1(In1)
  If/2 -> else/Action
  LOA_CNT_U08/1 -> If Action Subsystem1/1(In1)
  StOpCtrl_ScaleSV/1 -> If/2
  If/1 -> If Action Subsystem1/Action
  LoaScaleFctr/1 -> If/1, SelRampValue/1

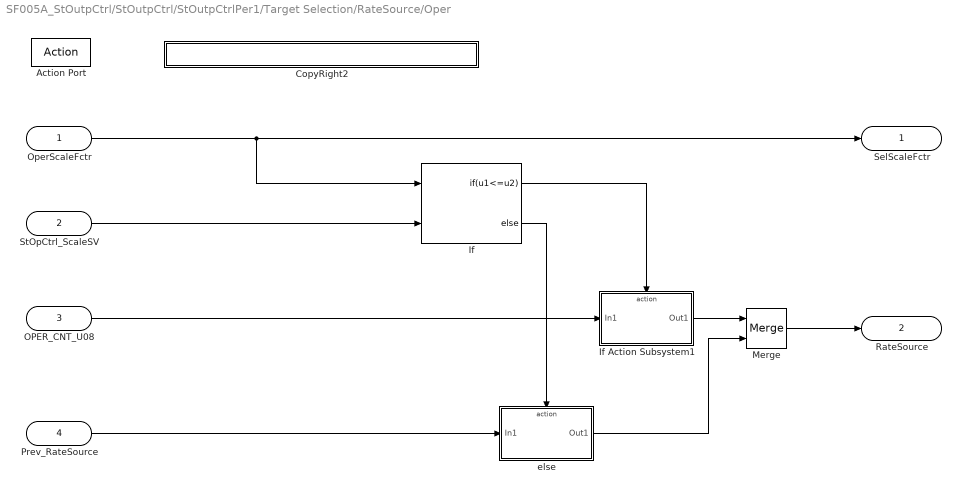
== system SF005A_StOutpCtrl/StOutpCtrl/StOutpCtrlPer1/Target Selection/RateSource/Oper ==
  OperScaleFctr : Inport
  StOpCtrl_ScaleSV : Inport  Port=2
  OPER_CNT_U08 : Inport  Port=3
  Prev_RateSource : Inport  Port=4
  Action Port : ActionPort  ActionType=case
  CopyRight2 : Subsystem  Description=|  mask(Copyright Information){none=on}
      | Copyright info block.                                               
      |                                                                     
      | Place copyright information at the top of every subsystem in design.
      mask prompts: none "No parameters"
      mask help: Place copyright information at the top of every subsystem in design.
      mask Display:
      | NxtrConf = 'Nexteer Confidential';
      | 
      | sys = bdroot; %handle for the current model ("system")
      | first = get_param(sys,'Created');
      | first = first(end-3:end);  %year is last four digits
      | 
      | last = get_param(sys,'LastModifiedDate');
      | if isempty(last)
      |     last = datestr(now,'yyyy');
      | else
      |     last = last(end-3:end);
      | end
      | 
      | if strcmp(first,last)
      |     fprintf('%s -- Copyright %s Nexteer',NxtrConf,first)
      | else
      |     fprintf('%s -- %s%s- %s Nexteer',NxtrConf,char(169),first,last)
      | end
  If : If  RequirementInfo={'linktype_rmi_doors' '0000baae (/E-STEER Core/SubSystem Specifications/Application Functions/SF005A State Output Control)' '#SF005A_54' 'true' 'REQ: SF005A_54' '' ; 'linktype_rmi_doors' '0000baae (/E-STEER Core/SubSystem Specifications/Application Functions/SF005A State Output Control)' '#SF005A_55' 'true' 'REQ: SF005A_55' '' ; 'linktype_rmi_doors' '0000baae (/E-STEER Core/SubSystem Specifications/Application Functions/SF005A State Output Control)' '#SF005A_61' 'true' 'REQ: SF005A_61' '' } %GIDa_7f0fcea9_e623_490b_b477_8070bf8ccca9  NumInputs=2  IfExpression=u1<=u2
  If Action Subsystem1 : Subsystem  TreatAsAtomicUnit=on
  Merge : Merge
  else : Subsystem  TreatAsAtomicUnit=on
  SelScaleFctr : Outport
  RateSource : Outport  Port=2
  wires:
  else/1(Out1) -> Merge/2
  If Action Subsystem1/1(Out1) -> Merge/1
  Merge/1 -> RateSource/1
  Prev_RateSource/1 -> else/1(In1)
  If/2 -> else/Action
  OPER_CNT_U08/1 -> If Action Subsystem1/1(In1)
  StOpCtrl_ScaleSV/1 -> If/2
  If/1 -> If Action Subsystem1/Action
  OperScaleFctr/1 -> If/1, SelScaleFctr/1

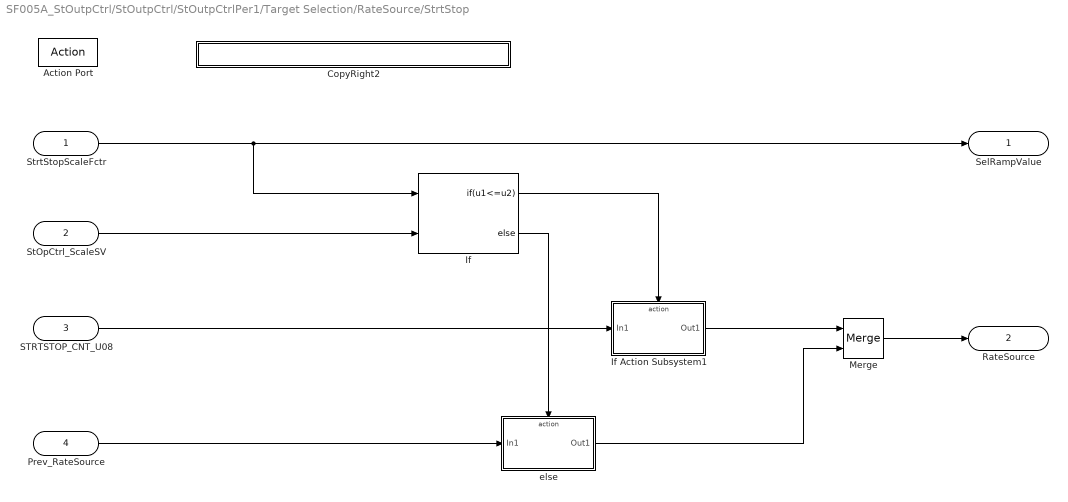
== system SF005A_StOutpCtrl/StOutpCtrl/StOutpCtrlPer1/Target Selection/RateSource/StrtStop ==
  StrtStopScaleFctr : Inport
  StOpCtrl_ScaleSV : Inport  Port=2
  STRTSTOP_CNT_U08 : Inport  Port=3
  Prev_RateSource : Inport  Port=4
  Action Port : ActionPort  ActionType=case
  CopyRight2 : Subsystem  Description=|  mask(Copyright Information){none=on}
      | Copyright info block.                                               
      |                                                                     
      | Place copyright information at the top of every subsystem in design.
      mask prompts: none "No parameters"
      mask help: Place copyright information at the top of every subsystem in design.
      mask Display:
      | NxtrConf = 'Nexteer Confidential';
      | 
      | sys = bdroot; %handle for the current model ("system")
      | first = get_param(sys,'Created');
      | first = first(end-3:end);  %year is last four digits
      | 
      | last = get_param(sys,'LastModifiedDate');
      | if isempty(last)
      |     last = datestr(now,'yyyy');
      | else
      |     last = last(end-3:end);
      | end
      | 
      | if strcmp(first,last)
      |     fprintf('%s -- Copyright %s Nexteer',NxtrConf,first)
      | else
      |     fprintf('%s -- %s%s- %s Nexteer',NxtrConf,char(169),first,last)
      | end
  If : If  RequirementInfo={'linktype_rmi_doors' '0000baae (/E-STEER Core/SubSystem Specifications/Application Functions/SF005A State Output Control)' '#SF005A_54' 'true' 'REQ: SF005A_54' '' ; 'linktype_rmi_doors' '0000baae (/E-STEER Core/SubSystem Specifications/Application Functions/SF005A State Output Control)' '#SF005A_55' 'true' 'REQ: SF005A_55' '' ; 'linktype_rmi_doors' '0000baae (/E-STEER Core/SubSystem Specifications/Application Functions/SF005A State Output Control)' '#SF005A_61' 'true' 'REQ: SF005A_61' '' } %GIDa_2d9fc241_76de_4798_baaf_ed414e6e2a48  NumInputs=2  IfExpression=u1<=u2
  If Action Subsystem1 : Subsystem  TreatAsAtomicUnit=on
  Merge : Merge
  else : Subsystem  TreatAsAtomicUnit=on
  SelRampValue : Outport
  RateSource : Outport  Port=2
  wires:
  else/1(Out1) -> Merge/2
  If Action Subsystem1/1(Out1) -> Merge/1
  Merge/1 -> RateSource/1
  Prev_RateSource/1 -> else/1(In1)
  If/2 -> else/Action
  StOpCtrl_ScaleSV/1 -> If/2
  If/1 -> If Action Subsystem1/Action
  StrtStopScaleFctr/1 -> If/1, SelRampValue/1
  STRTSTOP_CNT_U08/1 -> If Action Subsystem1/1(In1)

== system SF005A_StOutpCtrl/StOutpCtrl/StOutpCtrlPer1/Target Selection/RateSource/LOA/CopyRight2 ==

== system SF005A_StOutpCtrl/StOutpCtrl/StOutpCtrlPer1/Target Selection/RateSource/LOA/If Action Subsystem1 ==
  In1 : Inport
  Action Port : ActionPort  ActionType=then
  Out1 : Outport
  wires:
  In1/1 -> Out1/1
